simulink model "Simulacion_Control_Mandani_Sugeno"  (R2019a)
settings: Solver=VariableStepAuto  StartTime=0.0  StopTime=1000  RelTol=1e-3
libraries: fuzblock x2
settings Model: Creator=Alejoxbg  LastModifiedBy=Jose

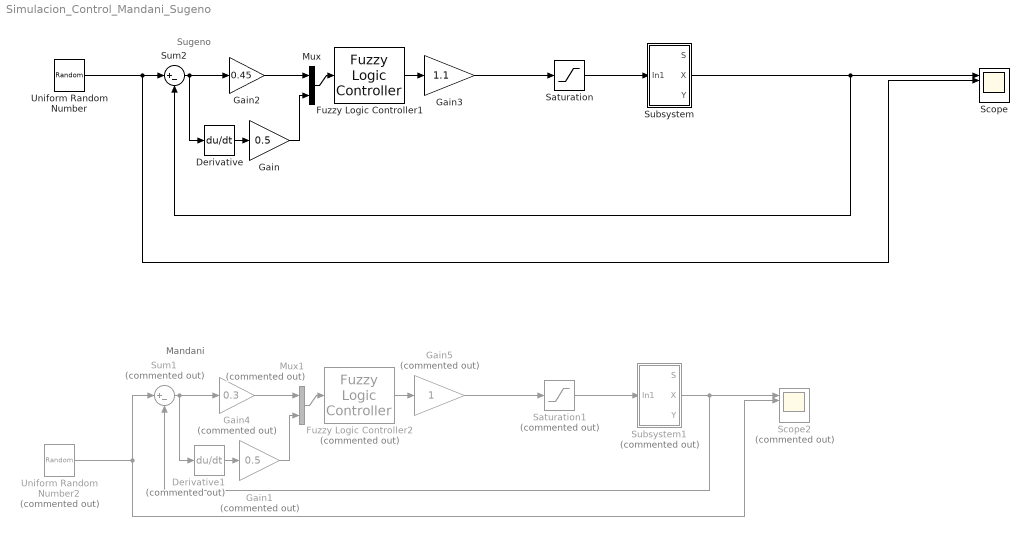
== system Simulacion_Control_Mandani_Sugeno ==
  note: Mandani
  note: Sugeno
  Derivative : Derivative
  Derivative1 : Derivative  Commented=on
  Fuzzy Logic Controller1 : fuzblock/Fuzzy Logic  Controller  FIS=fis  OutputSampleNumber=101  DataType=double  FuzzifiedInputs=off  RuleFiringStrengths=off  RuleOutputs=off  AggregatedOutputs=off  SimulateUsing=Interpreted execution  OutOfRangeInputValueMessage=warning  NoRuleFiredMessage=warning  EmptyOutputFuzzySetMessage=warning
  Fuzzy Logic Controller2 : fuzblock/Fuzzy Logic  Controller  Commented=on  FIS=fis  OutputSampleNumber=101  DataType=double  FuzzifiedInputs=off  RuleFiringStrengths=off  RuleOutputs=off  AggregatedOutputs=off  SimulateUsing=Interpreted execution  OutOfRangeInputValueMessage=warning  NoRuleFiredMessage=warning  EmptyOutputFuzzySetMessage=warning
  Gain : Gain  Gain=0.5
  Gain1 : Gain  Commented=on  Gain=0.5
  Gain2 : Gain  Gain=0.45
  Gain3 : Gain  Gain=1.1
  Gain4 : Gain  Commented=on  Gain=0.3
  Gain5 : Gain  Commented=on
  Mux : Mux  Inputs=2
  Mux1 : Mux  Commented=on  Inputs=2
  Saturation : Saturate  UpperLimit=1.7  LowerLimit=-1.7
  Saturation1 : Saturate  Commented=on  UpperLimit=1.7  LowerLimit=-1.7
  Scope : Scope  NumInputPorts=5
  Scope2 : Scope  Commented=on  NumInputPorts=5
  Subsystem : Subsystem
  Subsystem1 : Subsystem  Commented=on
  Sum1 : Sum  Commented=on  Inputs=|+-
  Sum2 : Sum  Inputs=|+-
  Uniform Random Number : UniformRandomNumber  Minimum=0.2  Seed=32  SampleTime=100
  Uniform Random Number2 : UniformRandomNumber  Commented=on  Minimum=0.2  Seed=32  SampleTime=100
  wires:
  Subsystem/2(X) -> Scope/1, Sum2/2
  Fuzzy Logic Controller1/1 -> Gain3/1
  Sum2/1 -> Derivative/1, Gain2/1
  Uniform Random Number/1 -> Scope/2, Sum2/1
  Mux/1 -> Fuzzy Logic Controller1/1
  Gain2/1 -> Mux/1
  Derivative/1 -> Gain/1
  Gain/1 -> Mux/2
  Gain3/1 -> Saturation/1
  Saturation/1 -> Subsystem/1(In1)
  Saturation1/1 -> Subsystem1/1(In1)
  Uniform Random Number2/1 -> Scope2/2, Sum1/1
  Derivative1/1 -> Gain1/1
  Mux1/1 -> Fuzzy Logic Controller2/1
  Gain4/1 -> Mux1/1
  Sum1/1 -> Derivative1/1, Gain4/1
  Gain1/1 -> Mux1/2
  Fuzzy Logic Controller2/1 -> Gain5/1
  Subsystem1/2(X) -> Scope2/1, Sum1/2
  Gain5/1 -> Saturation1/1

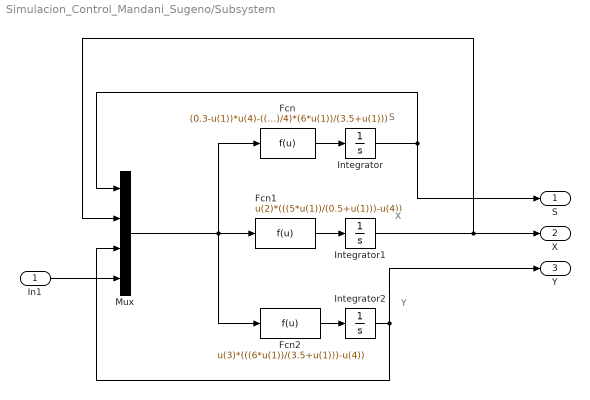
== system Simulacion_Control_Mandani_Sugeno/Subsystem ==
  note: X
  note: S
  note: Y
  In1 : Inport
  Fcn : Fcn  Expr=(0.3-u(1))*u(4)-((u(2)/4)*(5*u(1))/(0.5+u(1)))-((u(3)/4)*(6*u(1))/(3.5+u(1)))
  Fcn1 : Fcn  Expr=u(2)*(((5*u(1))/(0.5+u(1)))-u(4))
  Fcn2 : Fcn  Expr=u(3)*(((6*u(1))/(3.5+u(1)))-u(4))
  Integrator : Integrator
  Integrator1 : Integrator  InitialCondition=0.1
  Integrator2 : Integrator
  Mux : Mux
  S : Outport
  X : Outport  Port=2
  Y : Outport  Port=3
  wires:
  Fcn/1 -> Integrator/1
  Mux/1 -> Fcn/1, Fcn1/1, Fcn2/1
  Fcn2/1 -> Integrator2/1
  Integrator1/1 -> X/1, Mux/2
  Integrator2/1 -> Y/1, Mux/3
  Integrator/1 -> S/1, Mux/1
  In1/1 -> Mux/4
  Fcn1/1 -> Integrator1/1

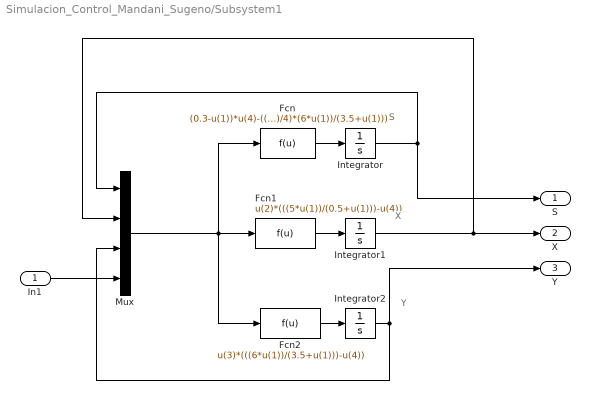
== system Simulacion_Control_Mandani_Sugeno/Subsystem1 ==
  note: X
  note: S
  note: Y
  In1 : Inport
  Fcn : Fcn  Expr=(0.3-u(1))*u(4)-((u(2)/4)*(5*u(1))/(0.5+u(1)))-((u(3)/4)*(6*u(1))/(3.5+u(1)))
  Fcn1 : Fcn  Expr=u(2)*(((5*u(1))/(0.5+u(1)))-u(4))
  Fcn2 : Fcn  Expr=u(3)*(((6*u(1))/(3.5+u(1)))-u(4))
  Integrator : Integrator
  Integrator1 : Integrator  InitialCondition=0.1
  Integrator2 : Integrator
  Mux : Mux
  S : Outport
  X : Outport  Port=2
  Y : Outport  Port=3
  wires:
  Fcn/1 -> Integrator/1
  Mux/1 -> Fcn/1, Fcn1/1, Fcn2/1
  Fcn2/1 -> Integrator2/1
  Integrator1/1 -> X/1, Mux/2
  Integrator2/1 -> Y/1, Mux/3
  Integrator/1 -> S/1, Mux/1
  In1/1 -> Mux/4
  Fcn1/1 -> Integrator1/1
